simulink model "E01"  (R2014a)
settings: Solver=ode45  StartTime=0.0  StopTime=40  RelTol=1e-3
libraries: cstblocks x2, simulink x1
settings Model: Creator=Davide  LastModifiedBy=Davide

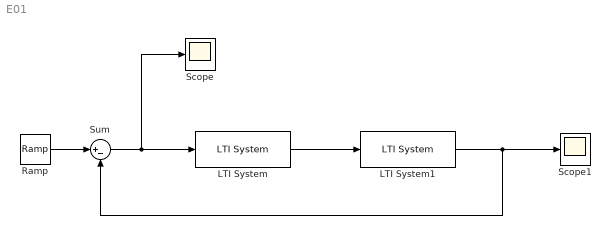
== system E01 ==
  LTI System : cstblocks/LTI System  sys=C  IC=[]
  LTI System1 : cstblocks/LTI System  sys=F1  IC=[]
  Ramp : simulink/Sources/Ramp  slope=1  start=0  X0=0
  Scope : Scope
  Scope1 : Scope
  Sum : Sum  Inputs=|+-
  wires:
  LTI System/1 -> LTI System1/1
  Ramp/1 -> Sum/1
  LTI System1/1 -> Sum/2, Scope1/1
  Sum/1 -> Scope/1, LTI System/1
